simulink model "test_8m_0508"  (R2024a)
settings: Solver=FixedStepAuto  StartTime=0.0  StopTime=30  FixedStep=dt  RelTol=1e-3
values from neighbouring files (symbols this model uses):
  attitude_0 = [0; -90;  -0]    [ini_param_8m_0522.m]
  b = 4.0    (= 4)    [ini_param_8m_0522.m]
  cbar = 0.75    [ini_param_8m_0522.m]
  dt = 0.004    [ini_param_8m_0522.m]
  H = 1000    [ini_param_8m_0522.m]
  N_data = [0,200, 491, 804, 1077, 1344, 1559, 1832, 2078, 2318, 2579,            2864, 3117, 3371, 3608.2, 3872, 4055.7, 4291, 4507, 4739, 4935]'    [cal_motor.m]
  N_pwm = 0.01*[0, 5 ,10 ,15 ,20 ,25 ,30 ,35,40, 45 ,50 ,              55 ,60 ,65 ,70, 75, 80 , 85 ,90 ,95 ,100]'    [cal_motor.m]
  pitch_rate_K = 1    [ini_param_8m_0522.m]
  roll_rate_K = 1    [ini_param_8m_0522.m]
  S = 6.0    (= 6)    [ini_param_8m_0522.m]
  Ts = 0.05    [ini_param_8m_0522.m]
  Ts_sur = 0.25    [ini_param_8m_0522.m]
  yaw_rate_K = 1    [ini_param_8m_0522.m]
undefined symbols (not defined in the file or in its folder): sigbuilder_block, UAV
libraries: slpidlib x9, simulink_extras x6, sharedtransform x2, shared6dof x1
(part 2 of 11)

== system test_8m_0508/速度控制/角速度环PID 需加限幅 ==
  note: 角速度环输出必须归一化
  r : Inport
  y : Inport  Port=2
  Add : Sum
  Constant : Constant  Value=[0;0;0]
  Demux1 : Demux  Outputs=3
  Demux2 : Demux  Outputs=3
  Gain : Gain  Gain=pitch_rate_K
  Gain1 : Gain  Gain=roll_rate_K
  Gain2 : Gain  Gain=yaw_rate_K
  MATLAB Function : MATLAB Function  TreatAsAtomicUnit=on
  Saturation : Saturate  UpperLimit=1  LowerLimit=-1
  Saturation1 : Saturate  UpperLimit=1  LowerLimit=-1
  Saturation2 : Saturate  UpperLimit=1  LowerLimit=-1
  Scope : Scope
  Scope1 : Scope
  Scope2 : Scope
  角加速度 : slpidlib/PID Controller (2DOF)  Controller=PID  Form=Parallel  TimeDomain=Discrete-time  UseExternalTs=off  SampleTime=0.004  IntegratorMethod=Forward Euler  FilterMethod=Forward Euler  ControllerParametersSource=internal  P=UAV.roll_rate_KP  I=UAV.roll_rate_KI  UseKiTs=off  D=UAV.roll_rate_KD  UseExternalDerivativeSource=off  N=100  UseFilter=on  b=1  c=0  TunerSelectOption=Transfer Function Based (PID Tuner App)  InitialConditionSource=internal  InitialConditionForIntegrator=0  InitialConditionForFilter=0  DifferentiatorICPrevScaledInput=0  ExternalReset=none  TrackingMode=off  Kt=1  LimitOutput=off  SatLimitsSource=internal  UpperSaturationLimit=UAV.pos_x.a_lim  LowerSaturationLimit=-UAV.pos_x.a_lim  LinearizeAsGain=on  AntiWindupMode=clamping  Kb=1  LimitIntegrator=off  UpperIntegratorSaturationLimit=inf  LowerIntegratorSaturationLimit=-inf  POutMin=[]  POutMax=[]  IOutMin=[]  IOutMax=[]  DOutMin=[]  DOutMax=[]  NOutMin=[]  NOutMax=[]  bOutMin=[]  bOutMax=[]  cOutMin=[]  cOutMax=[]  SumOutMin=[]  SumOutMax=[]  SaturationOutMin=[]  SaturationOutMax=[]  PParamMin=[]  PParamMax=[]  IParamMin=[]  IParamMax=[]  DParamMin=[]  DParamMax=[]  NParamMin=[]  NParamMax=[]  bParamMin=[]  bParamMax=[]  cParamMin=[]  cParamMax=[]  KbParamMin=[]  KbParamMax=[]  KtParamMin=[]  KtParamMax=[]  KbOutMin=[]  KbOutMax=[]  KtOutMin=[]  KtOutMax=[]  IntegratorOutMin=[]  IntegratorOutMax=[]  FilterOutMin=[]  FilterOutMax=[]  SumI1OutMin=[]  SumI1OutMax=[]  SumI2OutMin=[]  SumI2OutMax=[]  SumI3OutMin=[]  SumI3OutMax=[]  SumI4OutMin=[]  SumI4OutMax=[]  SumDOutMin=[]  SumDOutMax=[]  Sum1OutMin=[]  Sum1OutMax=[]  Sum2OutMin=[]  Sum2OutMax=[]  Sum3OutMin=[]  Sum3OutMax=[]  DifferentiatorOutMin=[]  DifferentiatorOutMax=[]  FilterDiffOutCoefMin=[]  FilterDiffOutCoefMax=[]  ReciprocalOutMin=[]  ReciprocalOutMax=[]  SumDenOutMin=[]  SumDenOutMax=[]  SumNumOutMin=[]  SumNumOutMax=[]  DivideOutMin=[]  DivideOutMax=[]  UdiffTsProdOutMin=[]  UdiffTsProdOutMax=[]  NTsProdOutMin=[]  NTsProdOutMax=[]  UintegralTsProdOutMin=[]  UintegralTsProdOutMax=[]  UngainTsProdOutMin=[]  UngainTsProdOutMax=[]  ClampingZeroOutDataTypeStr=Inherit: Inherit via back propagation  ClampingZeroOutMin=[]  ClampingZeroOutMax=[]  FilterDenConstantOutDataTypeStr=Inherit: Inherit via back propagation  FilterDenConstantOutMin=[]  FilterDenConstantOutMax=[]  PCopyOutDataTypeStr=Inherit: Inherit via back propagation  PCopyOutMin=[]  PCopyOutMax=[]  NCopyOutDataTypeStr=Inherit: Inherit via back propagation  NCopyOutMin=[]  NCopyOutMax=[]  IntegratorContinuousStateAttributes=''  IntegratorStateMustResolveToSignalObject=off  IntegratorRTWStateStorageClass=Auto  FilterContinuousStateAttributes=''  FilterStateMustResolveToSignalObject=off  FilterRTWStateStorageClass=Auto  ParallelPVariant=InternalParameters  IdealPVariant=Disabled  IVariant=InternalParameters  DVariant=InternalParameters  bVariant=InternalParameters  cVariant=InternalParameters  IntegratorVariant=Discrete  SatVariant=Disabled  AWVariant=Passthrough  PCopyVariant=Disabled  TRVariant=Disabled  FdbkBlocksVariant=Forward  IdealPFdbkVariant=Disabled  SatFdbkVariant=Disabled  DerivativeFilterVariant=ForwardEulerFilter  NVariant=InternalParameters  NCopyVariant=Disabled  FilterICVariant=InternalICsFilter  IntegratorICVariant=InternalICs  ExternalResetVariant=Disabled  TRSumVariant=Passthrough  SumFdbkVariant=Disabled  SumVariant=Sum_PID  TsampFilterVariant=InternalTs  TsampNgainVariant=Passthrough  TsampIntegralVariant=Disabled_SignalSpec  ExternalSaturationOutDataTypeStr=Inherit: Same as second input  DerivativeSourceVariant=ErrorSignal
  角加速度1 : slpidlib/PID Controller (2DOF)  Controller=PID  Form=Parallel  TimeDomain=Discrete-time  UseExternalTs=off  SampleTime=0.004  IntegratorMethod=Forward Euler  FilterMethod=Forward Euler  ControllerParametersSource=internal  P=UAV.pitch_rate_KP  I=UAV.pitch_rate_KI  UseKiTs=off  D=UAV.pitch_rate_KD  UseExternalDerivativeSource=off  N=100  UseFilter=on  b=1  c=0  TunerSelectOption=Transfer Function Based (PID Tuner App)  InitialConditionSource=internal  InitialConditionForIntegrator=0  InitialConditionForFilter=0  DifferentiatorICPrevScaledInput=0  ExternalReset=none  TrackingMode=off  Kt=1  LimitOutput=off  SatLimitsSource=external  UpperSaturationLimit=1  LowerSaturationLimit=-1  LinearizeAsGain=on  AntiWindupMode=clamping  Kb=1  LimitIntegrator=off  UpperIntegratorSaturationLimit=inf  LowerIntegratorSaturationLimit=-inf  POutMin=[]  POutMax=[]  IOutMin=[]  IOutMax=[]  DOutMin=[]  DOutMax=[]  NOutMin=[]  NOutMax=[]  bOutMin=[]  bOutMax=[]  cOutMin=[]  cOutMax=[]  SumOutMin=[]  SumOutMax=[]  SaturationOutMin=[]  SaturationOutMax=[]  PParamMin=[]  PParamMax=[]  IParamMin=[]  IParamMax=[]  DParamMin=[]  DParamMax=[]  NParamMin=[]  NParamMax=[]  bParamMin=[]  bParamMax=[]  cParamMin=[]  cParamMax=[]  KbParamMin=[]  KbParamMax=[]  KtParamMin=[]  KtParamMax=[]  KbOutMin=[]  KbOutMax=[]  KtOutMin=[]  KtOutMax=[]  IntegratorOutMin=[]  IntegratorOutMax=[]  FilterOutMin=[]  FilterOutMax=[]  SumI1OutMin=[]  SumI1OutMax=[]  SumI2OutMin=[]  SumI2OutMax=[]  SumI3OutMin=[]  SumI3OutMax=[]  SumI4OutMin=[]  SumI4OutMax=[]  SumDOutMin=[]  SumDOutMax=[]  Sum1OutMin=[]  Sum1OutMax=[]  Sum2OutMin=[]  Sum2OutMax=[]  Sum3OutMin=[]  Sum3OutMax=[]  DifferentiatorOutMin=[]  DifferentiatorOutMax=[]  FilterDiffOutCoefMin=[]  FilterDiffOutCoefMax=[]  ReciprocalOutMin=[]  ReciprocalOutMax=[]  SumDenOutMin=[]  SumDenOutMax=[]  SumNumOutMin=[]  SumNumOutMax=[]  DivideOutMin=[]  DivideOutMax=[]  UdiffTsProdOutMin=[]  UdiffTsProdOutMax=[]  NTsProdOutMin=[]  NTsProdOutMax=[]  UintegralTsProdOutMin=[]  UintegralTsProdOutMax=[]  UngainTsProdOutMin=[]  UngainTsProdOutMax=[]  ClampingZeroOutDataTypeStr=Inherit: Inherit via back propagation  ClampingZeroOutMin=[]  ClampingZeroOutMax=[]  FilterDenConstantOutDataTypeStr=Inherit: Inherit via back propagation  FilterDenConstantOutMin=[]  FilterDenConstantOutMax=[]  PCopyOutDataTypeStr=Inherit: Inherit via back propagation  PCopyOutMin=[]  PCopyOutMax=[]  NCopyOutDataTypeStr=Inherit: Inherit via back propagation  NCopyOutMin=[]  NCopyOutMax=[]  IntegratorContinuousStateAttributes=''  IntegratorStateMustResolveToSignalObject=off  IntegratorRTWStateStorageClass=Auto  FilterContinuousStateAttributes=''  FilterStateMustResolveToSignalObject=off  FilterRTWStateStorageClass=Auto  ParallelPVariant=InternalParameters  IdealPVariant=Disabled  IVariant=InternalParameters  DVariant=InternalParameters  bVariant=InternalParameters  cVariant=InternalParameters  IntegratorVariant=Discrete  SatVariant=Disabled  AWVariant=Passthrough  PCopyVariant=Disabled  TRVariant=Disabled  FdbkBlocksVariant=Forward  IdealPFdbkVariant=Disabled  SatFdbkVariant=Disabled  DerivativeFilterVariant=ForwardEulerFilter  NVariant=InternalParameters  NCopyVariant=Disabled  FilterICVariant=InternalICsFilter  IntegratorICVariant=InternalICs  ExternalResetVariant=Disabled  TRSumVariant=Passthrough  SumFdbkVariant=Disabled  SumVariant=Sum_PID  TsampFilterVariant=InternalTs  TsampNgainVariant=Passthrough  TsampIntegralVariant=Disabled_SignalSpec  ExternalSaturationOutDataTypeStr=Inherit: Same as second input  DerivativeSourceVariant=ErrorSignal
  角加速度2 : slpidlib/PID Controller (2DOF)  Controller=PID  Form=Parallel  TimeDomain=Discrete-time  UseExternalTs=off  SampleTime=0.004  IntegratorMethod=Forward Euler  FilterMethod=Forward Euler  ControllerParametersSource=internal  P=UAV.yaw_rate_KP  I=UAV.yaw_rate_KI  UseKiTs=off  D=UAV.yaw_rate_KD  UseExternalDerivativeSource=off  N=100  UseFilter=on  b=1  c=0  TunerSelectOption=Transfer Function Based (PID Tuner App)  InitialConditionSource=internal  InitialConditionForIntegrator=0  InitialConditionForFilter=0  DifferentiatorICPrevScaledInput=0  ExternalReset=none  TrackingMode=off  Kt=1  LimitOutput=off  SatLimitsSource=internal  UpperSaturationLimit=UAV.pos_z.a_lim  LowerSaturationLimit=-UAV.pos_z.a_lim  LinearizeAsGain=on  AntiWindupMode=clamping  Kb=UAV.v2acc.kb_z  LimitIntegrator=off  UpperIntegratorSaturationLimit=inf  LowerIntegratorSaturationLimit=-inf  POutMin=[]  POutMax=[]  IOutMin=[]  IOutMax=[]  DOutMin=[]  DOutMax=[]  NOutMin=[]  NOutMax=[]  bOutMin=[]  bOutMax=[]  cOutMin=[]  cOutMax=[]  SumOutMin=[]  SumOutMax=[]  SaturationOutMin=[]  SaturationOutMax=[]  PParamMin=[]  PParamMax=[]  IParamMin=[]  IParamMax=[]  DParamMin=[]  DParamMax=[]  NParamMin=[]  NParamMax=[]  bParamMin=[]  bParamMax=[]  cParamMin=[]  cParamMax=[]  KbParamMin=[]  KbParamMax=[]  KtParamMin=[]  KtParamMax=[]  KbOutMin=[]  KbOutMax=[]  KtOutMin=[]  KtOutMax=[]  IntegratorOutMin=[]  IntegratorOutMax=[]  FilterOutMin=[]  FilterOutMax=[]  SumI1OutMin=[]  SumI1OutMax=[]  SumI2OutMin=[]  SumI2OutMax=[]  SumI3OutMin=[]  SumI3OutMax=[]  SumI4OutMin=[]  SumI4OutMax=[]  SumDOutMin=[]  SumDOutMax=[]  Sum1OutMin=[]  Sum1OutMax=[]  Sum2OutMin=[]  Sum2OutMax=[]  Sum3OutMin=[]  Sum3OutMax=[]  DifferentiatorOutMin=[]  DifferentiatorOutMax=[]  FilterDiffOutCoefMin=[]  FilterDiffOutCoefMax=[]  ReciprocalOutMin=[]  ReciprocalOutMax=[]  SumDenOutMin=[]  SumDenOutMax=[]  SumNumOutMin=[]  SumNumOutMax=[]  DivideOutMin=[]  DivideOutMax=[]  UdiffTsProdOutMin=[]  UdiffTsProdOutMax=[]  NTsProdOutMin=[]  NTsProdOutMax=[]  UintegralTsProdOutMin=[]  UintegralTsProdOutMax=[]  UngainTsProdOutMin=[]  UngainTsProdOutMax=[]  ClampingZeroOutDataTypeStr=Inherit: Inherit via back propagation  ClampingZeroOutMin=[]  ClampingZeroOutMax=[]  FilterDenConstantOutDataTypeStr=Inherit: Inherit via back propagation  FilterDenConstantOutMin=[]  FilterDenConstantOutMax=[]  PCopyOutDataTypeStr=Inherit: Inherit via back propagation  PCopyOutMin=[]  PCopyOutMax=[]  NCopyOutDataTypeStr=Inherit: Inherit via back propagation  NCopyOutMin=[]  NCopyOutMax=[]  IntegratorContinuousStateAttributes=''  IntegratorStateMustResolveToSignalObject=off  IntegratorRTWStateStorageClass=Auto  FilterContinuousStateAttributes=''  FilterStateMustResolveToSignalObject=off  FilterRTWStateStorageClass=Auto  ParallelPVariant=InternalParameters  IdealPVariant=Disabled  IVariant=InternalParameters  DVariant=InternalParameters  bVariant=InternalParameters  cVariant=InternalParameters  IntegratorVariant=Discrete  SatVariant=Disabled  AWVariant=Passthrough  PCopyVariant=Disabled  TRVariant=Disabled  FdbkBlocksVariant=Forward  IdealPFdbkVariant=Disabled  SatFdbkVariant=Disabled  DerivativeFilterVariant=ForwardEulerFilter  NVariant=InternalParameters  NCopyVariant=Disabled  FilterICVariant=InternalICsFilter  IntegratorICVariant=InternalICs  ExternalResetVariant=Disabled  TRSumVariant=Passthrough  SumFdbkVariant=Disabled  SumVariant=Sum_PID  TsampFilterVariant=InternalTs  TsampNgainVariant=Passthrough  TsampIntegralVariant=Disabled_SignalSpec  ExternalSaturationOutDataTypeStr=Inherit: Same as second input  DerivativeSourceVariant=ErrorSignal
  accel_pid_out : Outport
  wires:
  Demux2/1 -> 角加速度/2
  r/1 -> Demux1/1
  y/1 -> Demux2/1
  Demux1/2 -> 角加速度1/1
  角加速度1/1 -> Gain/1
  Demux2/2 -> 角加速度1/2
  Demux2/3 -> 角加速度2/2
  Demux1/1 -> 角加速度/1
  角加速度2/1 -> Gain2/1
  角加速度/1 -> Gain1/1
  MATLAB Function/1(y) -> Add/1
  Constant/1 -> Add/2
  Add/1 -> accel_pid_out/1
  Demux1/3 -> 角加速度2/1
  Gain/1 -> Saturation1/1
  Gain1/1 -> Saturation/1
  Gain2/1 -> Saturation2/1
  Saturation/1 -> MATLAB Function/1(u1), Scope1/1
  Saturation1/1 -> Scope/1, MATLAB Function/2(u2)
  Saturation2/1 -> Scope2/1, MATLAB Function/3(u3)

== system test_8m_0508/速度控制/速度→加速度 需加限幅 ==
  r : Inport
  y : Inport  Port=2
  Add : Sum
  Constant : Constant  Value=[0;0;0]
  Demux1 : Demux  Outputs=3
  Demux2 : Demux  Outputs=3
  MATLAB Function : MATLAB Function  TreatAsAtomicUnit=on
  速度→加速度 : slpidlib/PID Controller (2DOF)  Controller=PID  Form=Parallel  TimeDomain=Discrete-time  UseExternalTs=off  SampleTime=0.004  IntegratorMethod=Forward Euler  FilterMethod=Forward Euler  ControllerParametersSource=internal  P=UAV.v2acc.kp_x  I=UAV.v2acc.ki_x  UseKiTs=off  D=UAV.v2acc.kd_x  UseExternalDerivativeSource=off  N=100  UseFilter=on  b=1  c=0  TunerSelectOption=Transfer Function Based (PID Tuner App)  InitialConditionSource=internal  InitialConditionForIntegrator=0  InitialConditionForFilter=0  DifferentiatorICPrevScaledInput=0  ExternalReset=none  TrackingMode=off  Kt=1  LimitOutput=on  SatLimitsSource=internal  UpperSaturationLimit=UAV.pos_x.a_lim  LowerSaturationLimit=-UAV.pos_x.a_lim  LinearizeAsGain=on  AntiWindupMode=clamping  Kb=1  LimitIntegrator=off  UpperIntegratorSaturationLimit=inf  LowerIntegratorSaturationLimit=-inf  POutMin=[]  POutMax=[]  IOutMin=[]  IOutMax=[]  DOutMin=[]  DOutMax=[]  NOutMin=[]  NOutMax=[]  bOutMin=[]  bOutMax=[]  cOutMin=[]  cOutMax=[]  SumOutMin=[]  SumOutMax=[]  SaturationOutMin=[]  SaturationOutMax=[]  PParamMin=[]  PParamMax=[]  IParamMin=[]  IParamMax=[]  DParamMin=[]  DParamMax=[]  NParamMin=[]  NParamMax=[]  bParamMin=[]  bParamMax=[]  cParamMin=[]  cParamMax=[]  KbParamMin=[]  KbParamMax=[]  KtParamMin=[]  KtParamMax=[]  KbOutMin=[]  KbOutMax=[]  KtOutMin=[]  KtOutMax=[]  IntegratorOutMin=[]  IntegratorOutMax=[]  FilterOutMin=[]  FilterOutMax=[]  SumI1OutMin=[]  SumI1OutMax=[]  SumI2OutMin=[]  SumI2OutMax=[]  SumI3OutMin=[]  SumI3OutMax=[]  SumI4OutMin=[]  SumI4OutMax=[]  SumDOutMin=[]  SumDOutMax=[]  Sum1OutMin=[]  Sum1OutMax=[]  Sum2OutMin=[]  Sum2OutMax=[]  Sum3OutMin=[]  Sum3OutMax=[]  DifferentiatorOutMin=[]  DifferentiatorOutMax=[]  FilterDiffOutCoefMin=[]  FilterDiffOutCoefMax=[]  ReciprocalOutMin=[]  ReciprocalOutMax=[]  SumDenOutMin=[]  SumDenOutMax=[]  SumNumOutMin=[]  SumNumOutMax=[]  DivideOutMin=[]  DivideOutMax=[]  UdiffTsProdOutMin=[]  UdiffTsProdOutMax=[]  NTsProdOutMin=[]  NTsProdOutMax=[]  UintegralTsProdOutMin=[]  UintegralTsProdOutMax=[]  UngainTsProdOutMin=[]  UngainTsProdOutMax=[]  ClampingZeroOutDataTypeStr=Inherit: Inherit via back propagation  ClampingZeroOutMin=[]  ClampingZeroOutMax=[]  FilterDenConstantOutDataTypeStr=Inherit: Inherit via back propagation  FilterDenConstantOutMin=[]  FilterDenConstantOutMax=[]  PCopyOutDataTypeStr=Inherit: Inherit via back propagation  PCopyOutMin=[]  PCopyOutMax=[]  NCopyOutDataTypeStr=Inherit: Inherit via back propagation  NCopyOutMin=[]  NCopyOutMax=[]  IntegratorContinuousStateAttributes=''  IntegratorStateMustResolveToSignalObject=off  IntegratorRTWStateStorageClass=Auto  FilterContinuousStateAttributes=''  FilterStateMustResolveToSignalObject=off  FilterRTWStateStorageClass=Auto  ParallelPVariant=InternalParameters  IdealPVariant=Disabled  IVariant=InternalParameters  DVariant=InternalParameters  bVariant=InternalParameters  cVariant=InternalParameters  IntegratorVariant=Discrete  SatVariant=Enabled  AWVariant=DiscClampingParallel  PCopyVariant=Disabled  TRVariant=Disabled  FdbkBlocksVariant=Forward  IdealPFdbkVariant=Disabled  SatFdbkVariant=Disabled  DerivativeFilterVariant=ForwardEulerFilter  NVariant=InternalParameters  NCopyVariant=Disabled  FilterICVariant=InternalICsFilter  IntegratorICVariant=InternalICs  ExternalResetVariant=Disabled  TRSumVariant=Passthrough  SumFdbkVariant=Disabled  SumVariant=Sum_PID  TsampFilterVariant=InternalTs  TsampNgainVariant=Passthrough  TsampIntegralVariant=Disabled_SignalSpec  ExternalSaturationOutDataTypeStr=Inherit: Same as second input  DerivativeSourceVariant=ErrorSignal
  速度→加速度1 : slpidlib/PID Controller (2DOF)  Controller=PID  Form=Parallel  TimeDomain=Discrete-time  UseExternalTs=off  SampleTime=0.004  IntegratorMethod=Forward Euler  FilterMethod=Forward Euler  ControllerParametersSource=internal  P=UAV.v2acc.kp_y  I=UAV.v2acc.ki_y  UseKiTs=off  D=UAV.v2acc.kd_y  UseExternalDerivativeSource=off  N=100  UseFilter=on  b=1  c=0  TunerSelectOption=Transfer Function Based (PID Tuner App)  InitialConditionSource=internal  InitialConditionForIntegrator=0  InitialConditionForFilter=0  DifferentiatorICPrevScaledInput=0  ExternalReset=none  TrackingMode=off  Kt=1  LimitOutput=on  SatLimitsSource=internal  UpperSaturationLimit=UAV.pos_y.a_lim  LowerSaturationLimit=-UAV.pos_y.a_lim  LinearizeAsGain=on  AntiWindupMode=clamping  Kb=1  LimitIntegrator=off  UpperIntegratorSaturationLimit=inf  LowerIntegratorSaturationLimit=-inf  POutMin=[]  POutMax=[]  IOutMin=[]  IOutMax=[]  DOutMin=[]  DOutMax=[]  NOutMin=[]  NOutMax=[]  bOutMin=[]  bOutMax=[]  cOutMin=[]  cOutMax=[]  SumOutMin=[]  SumOutMax=[]  SaturationOutMin=[]  SaturationOutMax=[]  PParamMin=[]  PParamMax=[]  IParamMin=[]  IParamMax=[]  DParamMin=[]  DParamMax=[]  NParamMin=[]  NParamMax=[]  bParamMin=[]  bParamMax=[]  cParamMin=[]  cParamMax=[]  KbParamMin=[]  KbParamMax=[]  KtParamMin=[]  KtParamMax=[]  KbOutMin=[]  KbOutMax=[]  KtOutMin=[]  KtOutMax=[]  IntegratorOutMin=[]  IntegratorOutMax=[]  FilterOutMin=[]  FilterOutMax=[]  SumI1OutMin=[]  SumI1OutMax=[]  SumI2OutMin=[]  SumI2OutMax=[]  SumI3OutMin=[]  SumI3OutMax=[]  SumI4OutMin=[]  SumI4OutMax=[]  SumDOutMin=[]  SumDOutMax=[]  Sum1OutMin=[]  Sum1OutMax=[]  Sum2OutMin=[]  Sum2OutMax=[]  Sum3OutMin=[]  Sum3OutMax=[]  DifferentiatorOutMin=[]  DifferentiatorOutMax=[]  FilterDiffOutCoefMin=[]  FilterDiffOutCoefMax=[]  ReciprocalOutMin=[]  ReciprocalOutMax=[]  SumDenOutMin=[]  SumDenOutMax=[]  SumNumOutMin=[]  SumNumOutMax=[]  DivideOutMin=[]  DivideOutMax=[]  UdiffTsProdOutMin=[]  UdiffTsProdOutMax=[]  NTsProdOutMin=[]  NTsProdOutMax=[]  UintegralTsProdOutMin=[]  UintegralTsProdOutMax=[]  UngainTsProdOutMin=[]  UngainTsProdOutMax=[]  ClampingZeroOutDataTypeStr=Inherit: Inherit via back propagation  ClampingZeroOutMin=[]  ClampingZeroOutMax=[]  FilterDenConstantOutDataTypeStr=Inherit: Inherit via back propagation  FilterDenConstantOutMin=[]  FilterDenConstantOutMax=[]  PCopyOutDataTypeStr=Inherit: Inherit via back propagation  PCopyOutMin=[]  PCopyOutMax=[]  NCopyOutDataTypeStr=Inherit: Inherit via back propagation  NCopyOutMin=[]  NCopyOutMax=[]  IntegratorContinuousStateAttributes=''  IntegratorStateMustResolveToSignalObject=off  IntegratorRTWStateStorageClass=Auto  FilterContinuousStateAttributes=''  FilterStateMustResolveToSignalObject=off  FilterRTWStateStorageClass=Auto  ParallelPVariant=InternalParameters  IdealPVariant=Disabled  IVariant=InternalParameters  DVariant=InternalParameters  bVariant=InternalParameters  cVariant=InternalParameters  IntegratorVariant=Discrete  SatVariant=Enabled  AWVariant=DiscClampingParallel  PCopyVariant=Disabled  TRVariant=Disabled  FdbkBlocksVariant=Forward  IdealPFdbkVariant=Disabled  SatFdbkVariant=Disabled  DerivativeFilterVariant=ForwardEulerFilter  NVariant=InternalParameters  NCopyVariant=Disabled  FilterICVariant=InternalICsFilter  IntegratorICVariant=InternalICs  ExternalResetVariant=Disabled  TRSumVariant=Passthrough  SumFdbkVariant=Disabled  SumVariant=Sum_PID  TsampFilterVariant=InternalTs  TsampNgainVariant=Passthrough  TsampIntegralVariant=Disabled_SignalSpec  ExternalSaturationOutDataTypeStr=Inherit: Same as second input  DerivativeSourceVariant=ErrorSignal
  速度→加速度2 : slpidlib/PID Controller (2DOF)  Controller=PID  Form=Parallel  TimeDomain=Discrete-time  UseExternalTs=off  SampleTime=0.004  IntegratorMethod=Forward Euler  FilterMethod=Forward Euler  ControllerParametersSource=internal  P=UAV.v2acc.kp_z  I=UAV.v2acc.ki_z  UseKiTs=off  D=UAV.v2acc.kd_z  UseExternalDerivativeSource=off  N=100  UseFilter=on  b=1  c=0  TunerSelectOption=Frequency Response Based  InitialConditionSource=internal  InitialConditionForIntegrator=0  InitialConditionForFilter=0  DifferentiatorICPrevScaledInput=0  ExternalReset=none  TrackingMode=off  Kt=1  LimitOutput=on  SatLimitsSource=internal  UpperSaturationLimit=UAV.pos_z.a_lim_up  LowerSaturationLimit=UAV.pos_z.a_lim_down  LinearizeAsGain=on  AntiWindupMode=clamping  Kb=UAV.v2acc.kb_z  LimitIntegrator=off  UpperIntegratorSaturationLimit=inf  LowerIntegratorSaturationLimit=-inf  POutMin=[]  POutMax=[]  IOutMin=[]  IOutMax=[]  DOutMin=[]  DOutMax=[]  NOutMin=[]  NOutMax=[]  bOutMin=[]  bOutMax=[]  cOutMin=[]  cOutMax=[]  SumOutMin=[]  SumOutMax=[]  SaturationOutMin=[]  SaturationOutMax=[]  PParamMin=[]  PParamMax=[]  IParamMin=[]  IParamMax=[]  DParamMin=[]  DParamMax=[]  NParamMin=[]  NParamMax=[]  bParamMin=[]  bParamMax=[]  cParamMin=[]  cParamMax=[]  KbParamMin=[]  KbParamMax=[]  KtParamMin=[]  KtParamMax=[]  KbOutMin=[]  KbOutMax=[]  KtOutMin=[]  KtOutMax=[]  IntegratorOutMin=[]  IntegratorOutMax=[]  FilterOutMin=[]  FilterOutMax=[]  SumI1OutMin=[]  SumI1OutMax=[]  SumI2OutMin=[]  SumI2OutMax=[]  SumI3OutMin=[]  SumI3OutMax=[]  SumI4OutMin=[]  SumI4OutMax=[]  SumDOutMin=[]  SumDOutMax=[]  Sum1OutMin=[]  Sum1OutMax=[]  Sum2OutMin=[]  Sum2OutMax=[]  Sum3OutMin=[]  Sum3OutMax=[]  DifferentiatorOutMin=[]  DifferentiatorOutMax=[]  FilterDiffOutCoefMin=[]  FilterDiffOutCoefMax=[]  ReciprocalOutMin=[]  ReciprocalOutMax=[]  SumDenOutMin=[]  SumDenOutMax=[]  SumNumOutMin=[]  SumNumOutMax=[]  DivideOutMin=[]  DivideOutMax=[]  UdiffTsProdOutMin=[]  UdiffTsProdOutMax=[]  NTsProdOutMin=[]  NTsProdOutMax=[]  UintegralTsProdOutMin=[]  UintegralTsProdOutMax=[]  UngainTsProdOutMin=[]  UngainTsProdOutMax=[]  ClampingZeroOutDataTypeStr=Inherit: Inherit via back propagation  ClampingZeroOutMin=[]  ClampingZeroOutMax=[]  FilterDenConstantOutDataTypeStr=Inherit: Inherit via back propagation  FilterDenConstantOutMin=[]  FilterDenConstantOutMax=[]  PCopyOutDataTypeStr=Inherit: Inherit via back propagation  PCopyOutMin=[]  PCopyOutMax=[]  NCopyOutDataTypeStr=Inherit: Inherit via back propagation  NCopyOutMin=[]  NCopyOutMax=[]  IntegratorContinuousStateAttributes=''  IntegratorStateMustResolveToSignalObject=off  IntegratorRTWStateStorageClass=Auto  FilterContinuousStateAttributes=''  FilterStateMustResolveToSignalObject=off  FilterRTWStateStorageClass=Auto  ParallelPVariant=InternalParameters  IdealPVariant=Disabled  IVariant=InternalParameters  DVariant=InternalParameters  bVariant=InternalParameters  cVariant=InternalParameters  IntegratorVariant=Discrete  SatVariant=Enabled  AWVariant=DiscClampingParallel  PCopyVariant=Disabled  TRVariant=Disabled  FdbkBlocksVariant=Forward  IdealPFdbkVariant=Disabled  SatFdbkVariant=Disabled  DerivativeFilterVariant=ForwardEulerFilter  NVariant=InternalParameters  NCopyVariant=Disabled  FilterICVariant=InternalICsFilter  IntegratorICVariant=InternalICs  ExternalResetVariant=Disabled  TRSumVariant=Passthrough  SumFdbkVariant=Disabled  SumVariant=Sum_PID  TsampFilterVariant=InternalTs  TsampNgainVariant=Passthrough  TsampIntegralVariant=Disabled_SignalSpec  ExternalSaturationOutDataTypeStr=Inherit: Same as second input  DerivativeSourceVariant=ErrorSignal
  accel_pid_out : Outport
  wires:
  Demux2/1 -> 速度→加速度/2
  r/1 -> Demux1/1
  y/1 -> Demux2/1
  Demux1/2 -> 速度→加速度1/1
  Demux2/2 -> 速度→加速度1/2
  Demux2/3 -> 速度→加速度2/2
  Demux1/1 -> 速度→加速度/1
  MATLAB Function/1(y) -> Add/1
  Constant/1 -> Add/2
  Add/1 -> accel_pid_out/1
  Demux1/3 -> 速度→加速度2/1
  速度→加速度2/1 -> MATLAB Function/3(u3)
  速度→加速度1/1 -> MATLAB Function/2(u2)
  速度→加速度/1 -> MATLAB Function/1(u1)

== system test_8m_0508/Aerodynamic_Model/Absolute Force&Moment/Subsystem1 ==
  rhoh : Inport
  TAS : Inport  Port=2
  Gain : Gain  Gain=1/2
  Product : Product
  Product1 : Product
  Square : Math  Operator=square
  WingArea : Constant  Value=S
  QS : Outport
  wires:
  TAS/1 -> Square/1
  Product/1 -> Product1/2  "Q"
  rhoh/1 -> Gain/1
  Gain/1 -> Product/1
  WingArea/1 -> Product1/1
  Product1/1 -> QS/1  "QS"
  Square/1 -> Product/2

== system test_8m_0508/Aerodynamic_Model/Co-efficent Calculation in wing FoR/CX_aero ==
  AeroCoeffients : Inport
  q : Inport  Port=2
  del_flap_rad : Inport  Port=3
  TAS : Inport  Port=4
  Add : Sum  Inputs=++++
  Add1 : Sum  Inputs=++++
  Bus Selector : BusSelector  OutputSignals=CD0,CD0_AF,CD_Q,CD_DF_FO,CD_DF_FI,CD_DF_RO,CD_DF_RI
  Demux : Demux
  Divide : Product  Inputs=*/
  Gain : Gain  Gain=cbar/2
  Gain1 : Gain  Gain=0.5
  Product{1..5} (5 alike) : Product
  CD : Outport
  wires:
  Add/1 -> CD/1  "CD"
  AeroCoeffients/1 -> Bus Selector/1
  Bus Selector/3 -> Product1/1  "<CD_Q>"
  TAS/1 -> Divide/2
  q/1 -> Gain/1
  Product1/1 -> Divide/1
  Bus Selector/1 -> Add/1  "<CD0>"
  Gain/1 -> Product1/2
  Divide/1 -> Add/3
  Bus Selector/2 -> Gain1/1  "<CD0_AF>"
  Gain1/1 -> Add/2
  del_flap_rad/1 -> Demux/1
  Bus Selector/4 -> Product2/1  "<CD_DF_FO>"
  Bus Selector/5 -> Product3/1  "<CD_DF_FI>"
  Bus Selector/6 -> Product4/1  "<CD_DF_RO>"
  Bus Selector/7 -> Product5/1  "<CD_DF_RI>"
  Product2/1 -> Add1/1
  Product3/1 -> Add1/2
  Product4/1 -> Add1/3
  Product5/1 -> Add1/4
  Demux/1 -> Product2/2
  Demux/2 -> Product3/2
  Demux/3 -> Product4/2
  Demux/4 -> Product5/2
  Add1/1 -> Add/4

== system test_8m_0508/Aerodynamic_Model/Co-efficent Calculation in wing FoR/CY_aero ==
  AeroCoeff : Inport
  beta : Inport  Port=2
  p : Inport  Port=3
  r : Inport  Port=4
  TAS : Inport  Port=5
  del_flap : Inport  Port=6
  del_alieron : Inport  Port=7
  Add : Sum  Inputs=+++++
  Add1 : Sum  Inputs=++++
  Add2 : Sum  Inputs=++++
  Bus Selector : BusSelector  OutputSignals=CS_B,CS_P,CS_R,CS_DA_FO,CS_DA_FI,CS_DA_RO,CS_DA_RI,CS_DF_FO,CS_DF_FI,CS_DF_RO,CS_DF_RI
  Demux : Demux
  Demux1 : Demux
  Divide : Product  Inputs=*/
  Divide1 : Product  Inputs=*/
  Gain : Gain  Gain=b/2
  Gain1 : Gain  Gain=b/2
  Product{,1..10} (11 alike) : Product
  CY : Outport
  wires:
  Add/1 -> CY/1  "CY"
  AeroCoeff/1 -> Bus Selector/1
  Bus Selector/1 -> Product/2  "<CS_B>"
  beta/1 -> Product/1
  Product/1 -> Add/1
  Bus Selector/2 -> Gain/1  "<CS_P>"
  Gain/1 -> Product1/1
  p/1 -> Product1/2
  Product1/1 -> Divide/1
  TAS/1 -> [TAS]
  [TAS] -> Divide/2
  Divide/1 -> Add/2
  Bus Selector/3 -> Gain1/1  "<CS_R>"
  Gain1/1 -> Product2/1
  r/1 -> Product2/2
  Product2/1 -> Divide1/1
  [TAS] -> Divide1/2
  Divide1/1 -> Add/3
  Bus Selector/4 -> Product3/1  "<CS_DA_FO>"
  Bus Selector/5 -> Product4/1  "<CS_DA_FI>"
  del_alieron/1 -> Demux/1
  del_flap/1 -> Demux1/1
  Bus Selector/6 -> Product5/1  "<CS_DA_RO>"
  Bus Selector/7 -> Product6/1  "<CS_DA_RI>"
  Bus Selector/8 -> Product7/1  "<CS_DF_FO>"
  Bus Selector/9 -> Product8/1  "<CS_DF_FI>"
  Bus Selector/10 -> Product9/1  "<CS_DF_RO>"
  Bus Selector/11 -> Product10/1  "<CS_DF_RI>"
  Demux/1 -> Product3/2
  Demux/2 -> Product4/2
  Demux/3 -> Product5/2
  Demux/4 -> Product6/2
  Demux1/1 -> Product7/2
  Demux1/2 -> Product8/2
  Demux1/3 -> Product9/2
  Demux1/4 -> Product10/2
  Product3/1 -> Add1/1
  Product4/1 -> Add1/2
  Product5/1 -> Add1/3
  Product6/1 -> Add1/4
  Product7/1 -> Add2/1
  Product8/1 -> Add2/2
  Product9/1 -> Add2/3
  Product10/1 -> Add2/4
  Add1/1 -> Add/4  "CY_aileron"
  Add2/1 -> Add/5  "CY_flap"

== system test_8m_0508/Aerodynamic_Model/Co-efficent Calculation in wing FoR/CZ_aero ==
  AeroCoeff : Inport
  q : Inport  Port=2
  del_flap : Inport  Port=3
  TAS : Inport  Port=4
  Add : Sum  Inputs=+++
  Add1 : Sum  Inputs=++++
  Bus Selector : BusSelector  OutputSignals=CL0,CL_Q,CL_DF_FO,CL_DF_FI,CL_DF_RO,CL_DF_RI
  Demux : Demux
  Divide : Product  Inputs=*/
  Gain : Gain  Gain=cbar/2
  Product{1,3..6} (5 alike) : Product
  CL : Outport
  wires:
  Add/1 -> CL/1  "CL"
  TAS/1 -> [TAS]
  AeroCoeff/1 -> Bus Selector/1
  Bus Selector/1 -> Add/1  "<CL0>"
  Bus Selector/2 -> Gain/1  "<CL_Q>"
  del_flap/1 -> Demux/1
  Gain/1 -> Product1/1
  q/1 -> Product1/2
  Product1/1 -> Divide/1
  [TAS] -> Divide/2
  Divide/1 -> Add/2
  Product4/1 -> Add1/2
  Product5/1 -> Add1/3
  Product6/1 -> Add1/4
  Product3/1 -> Add1/1
  Add1/1 -> Add/3  "CL_flap"
  Bus Selector/3 -> Product3/1  "<CL_DF_FO>"
  Bus Selector/4 -> Product4/1  "<CL_DF_FI>"
  Bus Selector/5 -> Product5/1  "<CL_DF_RO>"
  Bus Selector/6 -> Product6/1  "<CL_DF_RI>"
  Demux/1 -> Product3/2
  Demux/2 -> Product4/2
  Demux/3 -> Product5/2
  Demux/4 -> Product6/2

== system test_8m_0508/Aerodynamic_Model/Co-efficent Calculation in wing FoR/Cl_aero ==
  AeroCoeff : Inport
  beta : Inport  Port=2
  del_flap : Inport  Port=3
  del_alieron : Inport  Port=4
  p : Inport  Port=5
  r : Inport  Port=6
  TAS : Inport  Port=7
  Add : Sum  Inputs=+++++
  Add1 : Sum  Inputs=++++
  Add2 : Sum  Inputs=++++
  Bus Selector : BusSelector  OutputSignals=CLL_B,CLL_P,CLL_R,CLL_DA_FO,CLL_DA_FI,CLL_DA_RO,CLL_DA_RI,CLL_DF_FO,CLL_DF_FI,CLL_DF_RO,CLL_DF_RI
  Demux : Demux
  Demux1 : Demux
  Divide : Product  Inputs=*/
  Divide1 : Product  Inputs=*/
  Gain : Gain  Gain=b/2
  Gain1 : Gain  Gain=b/2
  Product{,1..10} (11 alike) : Product
  Scope{,1..5} (6 alike) : Scope
  Cl : Outport
  wires:
  Add/1 -> Scope5/1, Cl/1  "Cl"
  AeroCoeff/1 -> Bus Selector/1
  Bus Selector/1 -> Product/2  "<CLL_B>"
  beta/1 -> Product/1
  Bus Selector/2 -> Gain/1  "<CLL_P>"
  Gain/1 -> Product1/1
  p/1 -> Product1/2
  TAS/1 -> [TAS]
  Product1/1 -> Divide/1
  [TAS] -> Divide/2
  Bus Selector/3 -> Gain1/1  "<CLL_R>"
  Gain1/1 -> Product2/1
  r/1 -> Product2/2
  [TAS] -> Divide1/2
  Product2/1 -> Divide1/1
  Product/1 -> Scope2/1, Add/1
  Divide/1 -> Scope3/1, Add/2
  Divide1/1 -> Scope4/1, Add/3
  Product9/1 -> Add2/3
  Product8/1 -> Add2/2
  Product4/1 -> Add1/2
  Product7/1 -> Add2/1
  Product5/1 -> Add1/3
  Product6/1 -> Add1/4
  Product10/1 -> Add2/4
  Product3/1 -> Add1/1
  del_flap/1 -> Demux1/1
  del_alieron/1 -> Demux/1
  Add1/1 -> Scope1/1, Add/4  "Cl_aileron"
  Add2/1 -> Scope/1, Add/5  "Cl_flap"
  Bus Selector/4 -> Product3/1  "<CLL_DA_FO>"
  Bus Selector/5 -> Product4/1  "<CLL_DA_FI>"
  Bus Selector/6 -> Product5/1  "<CLL_DA_RO>"
  Bus Selector/7 -> Product6/1  "<CLL_DA_RI>"
  Demux/1 -> Product3/2
  Demux/2 -> Product4/2
  Demux/3 -> Product5/2
  Demux/4 -> Product6/2
  Bus Selector/8 -> Product7/1  "<CLL_DF_FO>"
  Bus Selector/9 -> Product8/1  "<CLL_DF_FI>"
  Bus Selector/10 -> Product9/1  "<CLL_DF_RO>"
  Bus Selector/11 -> Product10/1  "<CLL_DF_RI>"
  Demux1/1 -> Product7/2
  Demux1/2 -> Product8/2
  Demux1/3 -> Product9/2
  Demux1/4 -> Product10/2

== system test_8m_0508/Aerodynamic_Model/Co-efficent Calculation in wing FoR/Cm_aero ==
  AeroCoeff : Inport
  del_elevator : Inport  Port=2
  q : Inport  Port=3
  TAS : Inport  Port=4
  Add : Sum  Inputs=++++
  Add1 : Sum  Inputs=++++
  Bus Selector : BusSelector  OutputSignals=CM0,CM_AF,CM_Q,CM_DF_FO,CM_DF_FI,CM_DF_RO,CM_DF_RI
  Demux : Demux
  Divide : Product  Inputs=*/
  Gain : Gain  Gain=cbar/2
  Gain1 : Gain  Gain=0.5
  Product{,3..6} (5 alike) : Product
  Cm : Outport
  wires:
  Add/1 -> Cm/1  "Cm"
  AeroCoeff/1 -> Bus Selector/1
  Bus Selector/1 -> Add/1  "<CM0>"
  Gain/1 -> Product/1
  q/1 -> Product/2
  Product/1 -> Divide/1
  TAS/1 -> Divide/2
  del_elevator/1 -> Demux/1
  Demux/2 -> Product4/2
  Demux/3 -> Product5/2
  Product4/1 -> Add1/2
  Product6/1 -> Add1/4
  Product5/1 -> Add1/3
  Demux/1 -> Product3/2
  Demux/4 -> Product6/2
  Product3/1 -> Add1/1
  Bus Selector/3 -> Gain/1  "<CM_Q>"
  Divide/1 -> Add/3
  Add1/1 -> Add/4  "Cm_flap"
  Bus Selector/2 -> Gain1/1  "<CM_AF>"
  Gain1/1 -> Add/2
  Bus Selector/4 -> Product3/1  "<CM_DF_FO>"
  Bus Selector/5 -> Product4/1  "<CM_DF_FI>"
  Bus Selector/6 -> Product5/1  "<CM_DF_RO>"
  Bus Selector/7 -> Product6/1  "<CM_DF_RI>"

== system test_8m_0508/Aerodynamic_Model/Co-efficent Calculation in wing FoR/Cn_aero ==
  AeroCoeff : Inport
  beta : Inport  Port=2
  del_flap : Inport  Port=3
  del_alieoron : Inport  Port=4
  p : Inport  Port=5
  r : Inport  Port=6
  TAS : Inport  Port=7
  Add : Sum  Inputs=+++++
  Add1 : Sum  Inputs=++++
  Add2 : Sum  Inputs=++++
  Bus Selector : BusSelector  OutputSignals=CN_B,CN_P,CN_R,CN_DA_FO,CN_DA_FI,CN_DA_RO,CN_DA_RI,CN_DF_FO,CN_DF_FI,CN_DF_RO,CN_DF_RI
  Demux : Demux
  Demux1 : Demux
  Divide : Product  Inputs=*/
  Divide1 : Product  Inputs=*/
  Gain : Gain  Gain=b/2
  Gain1 : Gain  Gain=b/2
  Product{,1..2,6..13} (11 alike) : Product
  Cn : Outport
  wires:
  Add/1 -> Cn/1  "Cn"
  AeroCoeff/1 -> Bus Selector/1
  TAS/1 -> [TAS]
  Bus Selector/1 -> Product/1  "<CN_B>"
  beta/1 -> Product/2
  Product/1 -> Add/1
  Bus Selector/2 -> Gain/1  "<CN_P>"
  Gain/1 -> Product1/1
  p/1 -> Product1/2
  Product1/1 -> Divide/1
  [TAS] -> Divide/2
  Divide/1 -> Add/2
  Bus Selector/3 -> Gain1/1  "<CN_R>"
  Gain1/1 -> Product2/1
  r/1 -> Product2/2
  Product2/1 -> Divide1/1
  [TAS] -> Divide1/2
  Divide1/1 -> Add/3
  Demux1/1 -> Product11/2
  del_alieoron/1 -> Demux/1
  Demux1/4 -> Product10/2
  Demux/2 -> Product7/2
  Demux1/3 -> Product13/2
  Demux1/2 -> Product12/2
  del_flap/1 -> Demux1/1
  Product10/1 -> Add2/4
  Product7/1 -> Add1/2
  Product8/1 -> Add1/3
  Product12/1 -> Add2/2
  Product9/1 -> Add1/4
  Product6/1 -> Add1/1
  Demux/1 -> Product6/2
  Demux/3 -> Product8/2
  Demux/4 -> Product9/2
  Product11/1 -> Add2/1
  Product13/1 -> Add2/3
  Add1/1 -> Add/4  "Cn_aileron"
  Add2/1 -> Add/5  "Cn_flap"
  Bus Selector/4 -> Product6/1  "<CN_DA_FO>"
  Bus Selector/5 -> Product7/1  "<CN_DA_FI>"
  Bus Selector/6 -> Product8/1  "<CN_DA_RO>"
  Bus Selector/7 -> Product9/1  "<CN_DA_RI>"
  Bus Selector/8 -> Product11/1  "<CN_DF_FO>"
  Bus Selector/9 -> Product12/1  "<CN_DF_FI>"
  Bus Selector/10 -> Product13/1  "<CN_DF_RO>"
  Bus Selector/11 -> Product10/1  "<CN_DF_RI>"
